simulink model "Group_Component_1"  (R2024b)
settings: Solver=VariableStepAuto  StartTime=0.0  StopTime=20  MaxStep=0.0001  RelTol=1e-3
undefined symbols (not defined in the file): C, K1, K2, m1a, m1b, m2
settings Model: Creator=Noor Ur Rashid  LastModifiedBy=IMTIAZ AHMED

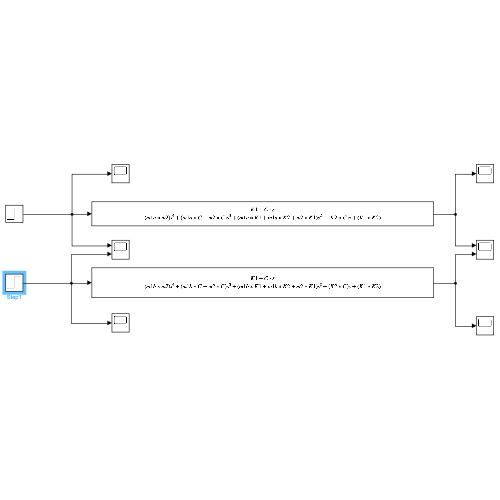
[thumbnail: Simulink's stored preview of the top-level diagram]
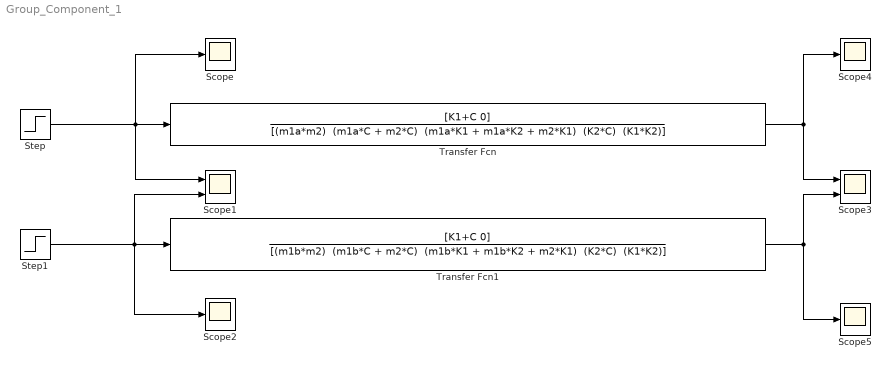
== system Group_Component_1 ==
  Scope{,2,4..5} (4 alike) : Scope
  Scope1 : Scope  NumInputPorts=2
  Scope3 : Scope  NumInputPorts=2
  Step : Step  After=m1a*9.80665*0.5  SampleTime=0
  Step1 : Step  After=m1b*9.80665*0.5  SampleTime=0
  Transfer Fcn : TransferFcn  Numerator=[K1+C 0]  Denominator="[(m1a*m2)  (m1a*C + m2*C)  (m1a*K1 + m1a*K2 + m2*K1)  (K2*C)  (K1*K2)]"
  Transfer Fcn1 : TransferFcn  Numerator=[K1+C 0]  Denominator="[(m1b*m2)  (m1b*C + m2*C)  (m1b*K1 + m1b*K2 + m2*K1)  (K2*C)  (K1*K2)]"
  wires:
  Step/1 -> Scope/1, Transfer Fcn/1, Scope1/1
  Step1/1 -> Scope2/1, Scope1/2, Transfer Fcn1/1
  Transfer Fcn1/1 -> Scope5/1, Scope3/2
  Transfer Fcn/1 -> Scope4/1, Scope3/1
